simulink model "qbot2"  (Simulink 7.7)
settings: Solver=FixedStepDiscrete  StartTime=0.0  StopTime=inf  FixedStep=0.005  RelTol=1e-3
undefined symbols (not defined in the file or in its folder): HIL
libraries: quarc_library x5, simulink_extras x1
settings Model: Creator=rhuq  LastModifiedBy=MT  SimulationMode=external  ExtModeTrigDuration=10000
settings SolverCC: PositivePriorityOrder=on
settings DataIOCC: SaveOutput=off  SaveTime=off
settings OptimizationCC: InitFltsAndDblsToZero=on
settings DebuggingCC: SaveWithParameterizedLinksMsg=none  InheritedTsInSrcMsg=none  MultiTaskDSMMsg=warning  MultiTaskCondExecSysMsg=none  StrictBusMsg=None
settings HardwareCC: TargetHWDeviceType=32-bit Generic
settings SFSimCC: SimParseCustomCode=off
settings RTWCC: SystemTargetFile=quarc_linux_verdex.tlc  TemplateMakefile=quarc_linux_arm_tmf  Description=QUARC Linux Verdex Target  ProcessScript=quarc_linux_verdex_make_rtw_hook  IncludeERTFirstTime=on
settings STFCustomTargetCC: TargetLibSuffix=.a  TargetPreCompLibLocation=C:\PROGRA~3\QUARC\lib\2011a\LINUX_~2\release  FunctionExecutionProfile=off  GeneratePreprocessorConditionals=Disable all  SystemTargetFile=quarc_linux_verdex.tlc
settings GRTTargetCC: TargetLibSuffix=.a  TargetPreCompLibLocation=C:\PROGRA~3\QUARC\lib\2011a\LINUX_~2\release  ParMdlRefBuildCompliant=off  CompOptLevelCompliant=off  MatFileLogging=off  ExtMode=on  ExtModeMexFile=quarc_comm  ExtModeMexArgs='-w -d /tmp -uri %u' 'tcpip://182.168.1.235:17001'
settings EnumStrPairs: String=LLVM-GCC

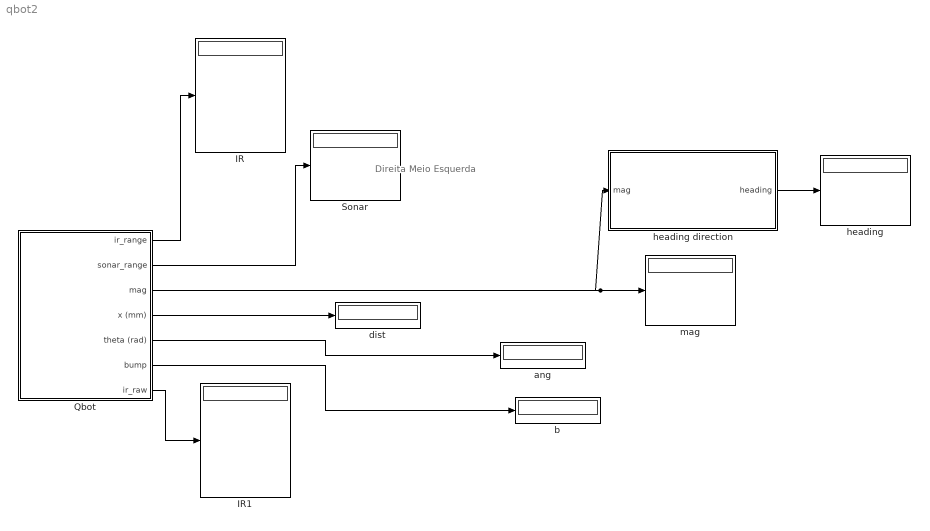
== system qbot2 ==
  note: Direita
      |
      | Meio
      |
      | Esquerda
  IR : Display
  IR1 : Display
  Qbot : Subsystem
  Sonar : Display
  ang : Display
  b : Display
  dist : Display
  heading : Display
  heading direction : Stateflow chart  TreatAsAtomicUnit=on
  mag : Display
  wires:
  Qbot/1(ir_range) -> IR/1
  Qbot/2(sonar_range) -> Sonar/1
  Qbot/3(mag) -> mag/1, heading direction/1(mag)
  Qbot/4(x (mm)) -> dist/1
  Qbot/5(theta (rad)) -> ang/1
  Qbot/6(bump) -> b/1
  Qbot/7(ir_raw) -> IR1/1
  heading direction/1(heading) -> heading/1

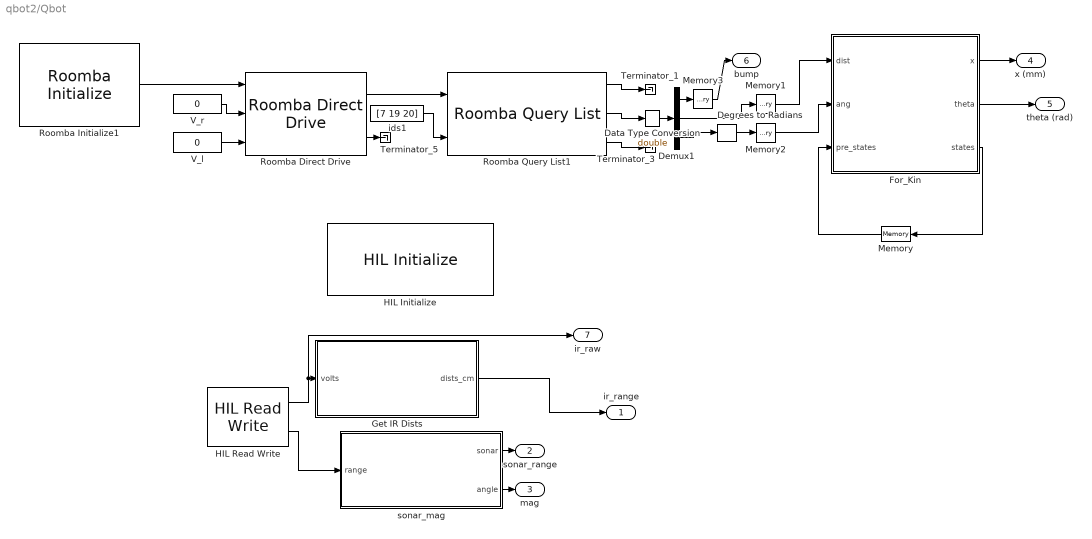
== system qbot2/Qbot ==
  Data Type Conversion : DataTypeConversion  OutDataTypeStr=double
  Degrees to Radians : simulink_extras/Transformations/Degrees to Radians  SystemSampleTime=-1
  Demux1 : Demux  Outputs=3
  For_Kin : Stateflow chart  TreatAsAtomicUnit=on
  Get IR Dists : Stateflow chart  TreatAsAtomicUnit=on
  HIL Initialize : quarc_library/Data Acquisition/Generic/Configuration/HIL Initialize  object_name=HIL-1  board_type=qbot  board_number=0  exclusive=off  active=on  hardware_clocks=[]  clock_modes=[]  initial_clock_frequencies=[]  set_clock_params_at_start=off  set_clock_params_at_switch_in=off  set_clock_frequencies_at_start=off  set_clock_frequencies_at_switch_in=off  analog_input_channels=[0:11]  analog_input_maximums=[]  analog_input_minimums=[]  set_analog_input_params_at_start=off  set_analog_input_params_at_switch_in=off  analog_output_channels=[]  analog_output_maximums=[]  analog_output_minimums=[]  initial_analog_outputs=[]  final_analog_outputs=[]  watchdog_analog_outputs=[]  set_analog_output_params_at_start=off  set_analog_output_params_at_switch_in=off  set_analog_outputs_at_start=off  set_analog_outputs_at_switch_in=off  set_analog_outputs_at_terminate=off  set_analog_outputs_at_switch_out=off  set_analog_outputs_on_watchdog=off  digital_input_channels=[]  digital_output_channels=[7]  digital_output_configuration=[]  initial_digital_outputs=[1]  final_digital_outputs=[1]  watchdog_digital_outputs=[]  set_digital_output_params_at_start=off  set_digital_output_params_at_switch_in=off  set_digital_outputs_at_start=on  set_digital_outputs_at_switch_in=off  set_digital_outputs_at_terminate=on  set_digital_outputs_at_switch_out=off  set_digital_outputs_on_watchdog=off  encoder_channels=[]  quadrature=[]  encoder_filter_frequency=[]  initial_encoder_counts=[]  set_encoder_params_at_start=off  set_encoder_params_at_switch_in=off  set_encoder_counts_at_start=off  set_encoder_counts_at_switch_in=off  pwm_channels=[0:7]  pwm_modes=[0]  pwm_frequency=50  pwm_configuration=[]  pwm_alignment=[]  pwm_polarity=[]  pwm_leading_deadband=[]  pwm_trailing_deadband=[]  initial_pwm_outputs=[0.075]  final_pwm_outputs=[0.075]  watchdog_pwm_outputs=[]  set_pwm_params_at_start=off  set_pwm_params_at_switch_in=off  set_pwm_outputs_at_start=on  set_pwm_outputs_at_switch_in=off  set_pwm_outputs_at_terminate=on  set_pwm_outputs_at_switch_out=off  set_pwm_outputs_on_watchdog=off  other_output_channels=[]  initial_other_outputs=[]  final_other_outputs=[]  watchdog_other_outputs=[]  set_other_outputs_at_start=off  set_other_outputs_at_switch_in=off  set_other_outputs_at_terminate=off  set_other_outputs_at_switch_out=off  set_other_outputs_on_watchdog=off
  HIL Read Write : quarc_library/Data Acquisition/Generic/Immediate I//O/HIL Read Write  object_name=HIL-1  analog_output_channels=[]  pwm_output_channels=[]  digital_output_channels=[]  other_output_channels=[]  analog_input_channels=[7:11]  encoder_input_channels=[]  digital_input_channels=[]  other_input_channels=[3:5 8000:8002]  sample_time=qc_get_step_size  active=off  vector_output=on  vector_input=off  data_type_mode=Inherit via back propagation  encoder_data_type=double  digital_data_type=boolean
      settings: AttributesFormatString=(%<object_name>)
  Memory : Memory  X0=[0 0 0 0]
  Memory1 : Memory
  Memory2 : Memory
  Memory3 : Memory
  Roomba Direct Drive : quarc_library/Devices/Third-Party/iRobot/Roomba/Interfacing/Roomba Direct Drive  sample_time=qc_get_step_size
  Roomba Initialize1 : quarc_library/Devices/Third-Party/iRobot/Roomba/Interfacing/Roomba Initialize  uri=serial://localhost:1?baud=57600,word=8,parity=none,stop=1  send_buffer_size=100  receive_buffer_size=100  active=off
  Roomba Query List1 : quarc_library/Devices/Third-Party/iRobot/Roomba/Interfacing/Roomba Query List  sample_time=qc_get_step_size
  Terminator_1 : Terminator
  Terminator_3 : Terminator
  Terminator_5 : Terminator
  V_l : Constant  Value=0  OutDataTypeStr=Inherit: Inherit via back propagation
  V_r : Constant  Value=0  OutDataTypeStr=Inherit: Inherit via back propagation
  ids1 : Constant  Value=[7 19 20]  OutDataTypeStr=Inherit: Inherit via back propagation
  sonar_mag : Stateflow chart  TreatAsAtomicUnit=on
  ir_range : Outport
  sonar_range : Outport  Port=2
  mag : Outport  Port=3
  x (mm) : Outport  Port=4
  theta (rad) : Outport  Port=5
  bump : Outport  Port=6
  ir_raw : Outport  Port=7
  wires:
  HIL Read Write/2 -> sonar_mag/1(range)
  sonar_mag/1(sonar) -> sonar_range/1
  sonar_mag/2(angle) -> mag/1
  Roomba Initialize1/1 -> Roomba Direct Drive/1
  Roomba Direct Drive/2 -> Terminator_5/1
  Roomba Direct Drive/1 -> Roomba Query List1/1
  ids1/1 -> Roomba Query List1/2
  V_r/1 -> Roomba Direct Drive/2
  V_l/1 -> Roomba Direct Drive/3
  Degrees to Radians/1 -> Memory2/1
  Data Type Conversion/1 -> Demux1/1
  Demux1/1 -> Memory3/1
  Demux1/2 -> Memory1/1
  Demux1/3 -> Degrees to Radians/1
  Memory3/1 -> bump/1
  Roomba Query List1/1 -> Terminator_1/1
  Roomba Query List1/2 -> Data Type Conversion/1
  Roomba Query List1/3 -> Terminator_3/1
  For_Kin/3(states) -> Memory/1
  Memory/1 -> For_Kin/3(pre_states)
  Memory1/1 -> For_Kin/1(dist)
  Memory2/1 -> For_Kin/2(ang)
  For_Kin/1(x) -> x (mm)/1
  For_Kin/2(theta) -> theta (rad)/1
  HIL Read Write/1 -> Get IR Dists/1(volts), ir_raw/1
  Get IR Dists/1(dists_cm) -> ir_range/1

== matlab function Qbot/sonar_mag ==
  data: range input double; sonar output double; angle output double
function [sonar,angle]  = read_data(range)
sonar=range(1:3);
angle=range(4:6)*100;
return

== matlab function heading direction ==
  data: mag input double; heading output double
function heading  = heading_direction(mag)
magx=-41.956587966488950;
magy=13.730769230769230;
heading=mod(atan2(mag(1)-magx,mag(2)-magy)*180/pi,360);
return;

== matlab function Qbot/For_Kin ==
  data: dist input double; x output double; ang input double; pre_states input double; theta output double; states output double
function [x, theta, states] = for_kin(dist, ang, pre_states)
% This block supports an embeddable subset of the MATLAB language.
% See the help menu for details. 

states = pre_states;

if states(1) == 0
    x = 0;
    theta = 0;
    states(1) = 1;
else
    x = states(2) + dist;
    theta = check_angle(check_angle(states(3)) + check_angle(ang));
end

states(2) = x;
states(3) = theta;

return;

function y = check_angle(x)
y = x;
if y > pi
    y = x - 2*pi;
elseif y < -pi
    y = x + 2*pi;
end
return;

== matlab function Qbot/Get IR Dists ==
  data: volts input double; dists_cm output double
function dists_cm  = get_ir_dists(volts)
% This block supports the Embedded MATLAB subset.
% See the help menu for details. 


rlimit = 1.50; % 150 cm
%C=[0.0526 -0.4859 1.8328 -3.6110 3.9039 -2.1333 0.3226 0.1746];
C=[-18.4153  147.1579 -450.3636  632.0092 -319.7520 -141.5864  210.4675];
%C=[-18.41533900452932926 147.1579026586913983 -450.3635939931881467 632.0091740249222312 -319.7520456770031956 -141.5863628740575280 210.4674822778460168];
%C = [3.7354  -47.8837  193.7820 -333.2112  239.9496];
dists_cm = polyval(C, volts)/100;
%dists_cm(volts>2.6)=0.2;
% n = length(dists_cm);
% 
% for i=1:n
%     if dists_cm(i)<0.20
%         dists_cm(i) = 0;
%     end
%     if dists_cm(i)>rlimit
%         dists_cm(i) = rlimit+0.01;
%     end
% end

return;
